simulink model "speed_control_for_IM"  (R2021a)
settings: Solver=VariableStepAuto  StartTime=0.0  StopTime=inf  MaxStep=1e-3  RelTol=1e-3
libraries: spsIGBTDiodeLib x6, spsAsynchronousMachineSIUnitsLib x1, pid_lib x1, spsDCVoltageSourceLib x1, simulink x1, spspowerguiLib x1
settings Model: Creator=AHMED  LastModifiedBy=AHMED

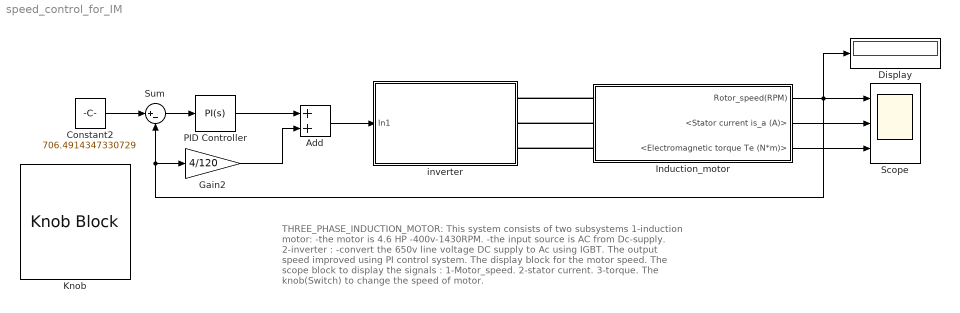
== system speed_control_for_IM ==
  note: THREE_PHASE_INDUCTION_MOTOR:
      |
      | This system consists of two subsystems
      | 1-induction motor:
      | -the motor is 4.6 HP -400v-1430RPM.
      | -the input source is AC from Dc-supply.
      | 2-inverter :
      | -convert the 650v line voltage DC supply to Ac using IGBT.
      |
      | The output speed improved using PI control system.
      | The display block for the motor speed.
      | The scope block to display the signals :
      | 1-Motor_speed.
      | 2-stator current.
      | 3-torque.
      | The knob(Switch) to change the speed of motor.
  Add : Sum
  Constant2 : Constant  Value=706.4914347330729
  Display : Display
  Gain2 : Gain  Gain=4/120
  Induction_motor : Subsystem
  Knob : KnobBlock  ScaleMax=1400
  PID Controller : pid_lib/PID Controller  Controller=PI  Form=Parallel  TimeDomain=Continuous-time  UseExternalTs=off  SampleTime=-1  IntegratorMethod=Forward Euler  FilterMethod=Forward Euler  ControllerParametersSource=internal  P=1.5  I=0.001  D=0  UseFilter=on  N=100  TunerSelectOption=Transfer Function Based (PID Tuner App)  InitialConditionSource=internal  InitialConditionForIntegrator=0  InitialConditionForFilter=0  DifferentiatorICPrevScaledInput=0  ExternalReset=none  TrackingMode=off  Kt=1  LimitOutput=on  SatLimitsSource=internal  UpperSaturationLimit=50  LowerSaturationLimit=-50  LinearizeAsGain=on  AntiWindupMode=clamping  Kb=1  POutMin=[]  POutMax=[]  IOutMin=[]  IOutMax=[]  DOutMin=[]  DOutMax=[]  NOutMin=[]  NOutMax=[]  SumOutMin=[]  SumOutMax=[]  SaturationOutMin=[]  SaturationOutMax=[]  PParamMin=[]  PParamMax=[]  IParamMin=[]  IParamMax=[]  DParamMin=[]  DParamMax=[]  NParamMin=[]  NParamMax=[]  KbParamMin=[]  KbParamMax=[]  KtParamMin=[]  KtParamMax=[]  KbOutMin=[]  KbOutMax=[]  KtOutMin=[]  KtOutMax=[]  IntegratorOutMin=[]  IntegratorOutMax=[]  FilterOutMin=[]  FilterOutMax=[]  SumI1OutMin=[]  SumI1OutMax=[]  SumI2OutMin=[]  SumI2OutMax=[]  SumI3OutMin=[]  SumI3OutMax=[]  SumI4OutMin=[]  SumI4OutMax=[]  SumDOutMin=[]  SumDOutMax=[]  DifferentiatorOutMin=[]  DifferentiatorOutMax=[]  FilterDiffOutCoefMin=[]  FilterDiffOutCoefMax=[]  ReciprocalOutMin=[]  ReciprocalOutMax=[]  SumDenOutMin=[]  SumDenOutMax=[]  SumNumOutMin=[]  SumNumOutMax=[]  DivideOutMin=[]  DivideOutMax=[]  UdiffTsProdOutMin=[]  UdiffTsProdOutMax=[]  NTsProdOutMin=[]  NTsProdOutMax=[]  UintegralTsProdOutMin=[]  UintegralTsProdOutMax=[]  UngainTsProdOutMin=[]  UngainTsProdOutMax=[]  IntegratorContinuousStateAttributes=''  IntegratorStateMustResolveToSignalObject=off  IntegratorRTWStateStorageClass=Auto  FilterContinuousStateAttributes=''  FilterStateMustResolveToSignalObject=off  FilterRTWStateStorageClass=Auto  ParallelPVariant=InternalParameters  IdealPVariant=Disabled  IVariant=InternalParameters  DVariant=Disabled  IntegratorVariant=Continuous  SatVariant=Enabled  AWVariant=ContClampingParallel  PCopyVariant=Disabled  TRVariant=Disabled  FdbkBlocksVariant=Forward  IdealPFdbkVariant=Disabled  SatFdbkVariant=Disabled  DerivativeFilterVariant=Disabled  NVariant=Disabled  NCopyVariant=Disabled_SignalSpec  FilterICVariant=Disabled  IntegratorICVariant=InternalICs  ExternalResetVariant=Disabled  TRSumVariant=Passthrough  SumFdbkVariant=Disabled  SumVariant=Sum_PI  TsampFilterVariant=InternalTs  TsampNgainVariant=Passthrough  TsampIntegralVariant=Passthrough  ExternalSaturationOutDataTypeStr=Inherit: Same as second input
  Scope : Scope  NumInputPorts=3
  Sum : Sum  Inputs=|+-
  inverter : Subsystem
  wires:
  Sum/1 -> PID Controller/1
  Constant2/1 -> Sum/1
  PID Controller/1 -> Add/1
  Gain2/1 -> Add/2
  Induction_motor/1(Rotor_speed(RPM)) -> Gain2/1, Sum/2, Scope/1, Display/1
  Induction_motor/2(<Stator current is_a (A)>) -> Scope/2
  Induction_motor/3(<Electromagnetic torque Te (N*m)>) -> Scope/3
  Add/1 -> inverter/1(In1)
  connections:
  Induction_motor/LConn1 -- inverter/RConn1
  Induction_motor/LConn2 -- inverter/RConn2
  Induction_motor/LConn3 -- inverter/RConn3

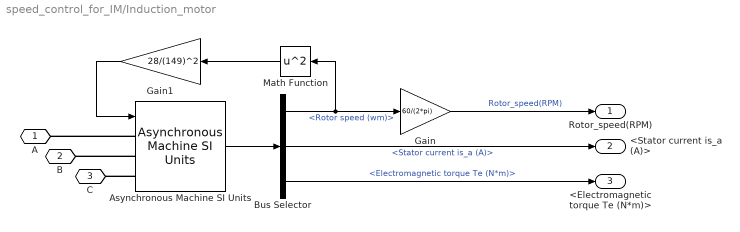
== system speed_control_for_IM/Induction_motor ==
  Asynchronous Machine SI Units : spsAsynchronousMachineSIUnitsLib/Asynchronous Machine SI Units  RotorType=Squirrel-cage  PresetModel="15:  5.4 HP (4KW)   400 V  50Hz 1430 RPM"  MechanicalLoad=Torque Tm  ShowDetailedParameters=on  ReferenceFrame=Rotor  Units=SI  MeasurementBus=off  NominalParameters=[4000 400 50]  VoltageRatio=1  Stator=[1.405 0.005839]  Rotor=[1.395 0.005839]  Cage1=[0.4155 0.002066]  Cage2=[0.4168 0.0003495]  Lm=0.1722  Mechanical=[0.0131 0.002985 2]  PolePairs=2  InitialConditions=[1 0 0 0 0 0 0 0]  SimulateSaturation=off  Saturation=[14.03593122, 27.81365428, 53.79336849, 72.68890987, 97.98006896, 148.6815601, 215.7428561, 302.9841135, 428.7778367 ; 230, 322, 414, 460, 506, 552, 598, 644, 690]  LoadFlowParameters=1492000  TsPowergui=0  TsBlock=-1  IterativeModel=Trapezoidal non iterative  IterativeDiscreteModel=Trapezoidal non iterative  Pmec=1.492e+006
  Bus Selector : BusSelector  OutputSignals=Mechanical.Rotor speed (wm),Stator measurements.Stator current is_a (A),Mechanical.Electromagnetic torque Te (N*m)
  Gain : Gain  Gain=60/(2*pi)
  Gain1 : Gain  Gain=28/(149)^2
  Math Function : Math  Operator=square  SaturateOnIntegerOverflow=on
  A : PMIOPort  Side=Left
  B : PMIOPort  Port=2  Side=Left
  C : PMIOPort  Port=3  Side=Left
  Rotor_speed(RPM) : Outport
  <Stator current is_a (A)> : Outport  Port=2
  <Electromagnetic torque Te (N*m)> : Outport  Port=3
  wires:
  Gain/1 -> Rotor_speed(RPM)/1  "Rotor_speed(RPM)"
  Bus Selector/1 -> Math Function/1, Gain/1  "<Rotor speed (wm)>"
  Bus Selector/3 -> <Electromagnetic torque Te (N*m)>/1  "<Electromagnetic torque Te (N*m)>"
  Bus Selector/2 -> <Stator current is_a (A)>/1  "<Stator current is_a (A)>"
  Asynchronous Machine SI Units/1 -> Bus Selector/1
  Gain1/1 -> Asynchronous Machine SI Units/1
  Math Function/1 -> Gain1/1
  connections:
  Asynchronous Machine SI Units/LConn1 -- A/RConn1
  Asynchronous Machine SI Units/LConn2 -- B/RConn1
  Asynchronous Machine SI Units/LConn3 -- C/RConn1

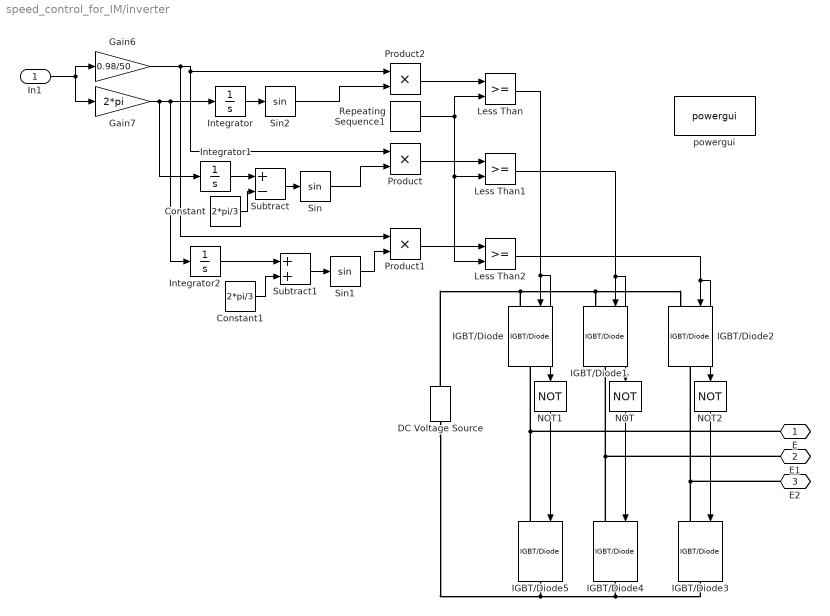
== system speed_control_for_IM/inverter ==
  In1 : Inport
  Constant : Constant  Value=2*pi/3
  Constant1 : Constant  Value=2*pi/3
  DC Voltage Source : spsDCVoltageSourceLib/DC Voltage Source  Amplitude=650  Measurements=None
  Gain6 : Gain  Gain=0.98/50
  Gain7 : Gain  Gain=2*pi
  IGBT/Diode{,1..5} (6 alike) : spsIGBTDiodeLib/IGBT//Diode  Ron=1e-3  Rs=1e5  Cs=inf  Measurements=off
  Integrator : Integrator
  Integrator1 : Integrator
  Integrator2 : Integrator
  Less Than : RelationalOperator  OutDataTypeStr=boolean  RndMeth=Simplest
  Less Than1 : RelationalOperator  OutDataTypeStr=boolean  RndMeth=Simplest
  Less Than2 : RelationalOperator  OutDataTypeStr=boolean  RndMeth=Simplest
  NOT : Logic  Operator=NOT  AllPortsSameDT=off  OutDataTypeStr=boolean
  NOT1 : Logic  Operator=NOT  AllPortsSameDT=off  OutDataTypeStr=boolean
  NOT2 : Logic  Operator=NOT  AllPortsSameDT=off  OutDataTypeStr=boolean
  Product : Product
  Product1 : Product
  Product2 : Product
  Repeating Sequence1 : simulink/Sources/Repeating Sequence  rep_seq_t=[0 (1/5000)/4 (1/5000)/2 (3/5000)/4 1/5000]  rep_seq_y=[0 1 0 -1 0]
  Sin : Trigonometry
  Sin1 : Trigonometry
  Sin2 : Trigonometry
  Subtract : Sum  Inputs=+-
  Subtract1 : Sum
  powergui : spspowerguiLib/powergui  Priority=1  SimulationMode=Discrete  SampleTime=1e-6  frequency=60  Iterations=50  frequencyindice=50  Pbase=100e6  ErrMax=1e-4  UnitsV=kV  UnitsW=MW  buscounter=0  FunctionMessages=off  echomessages=off  EnableUseOfTLC=off  CurrentSourceSwitches=off  DisableSnubberDevices=off  DisableRonSwitches=off  DisableVfSwitches=off  DisplayEquations=off  AutomaticDiscreteSolvers=off  SolverType=Tustin/Backward Euler (TBE)  Interpol=off  ExternalGateDelay=off  methode=off  Ts=100  x0status=blocks  SPID=on  SwTol=0  HookPort=off  NonlinearTolerance=1e-4  nMaxIteration=100  ContinueOnMaxIteration=off  RestoreLinks=warning  ResistiveCurrentMeasurement=off  Frange=[0:2:500]  Ylog=off  Xlog=on  ShowGrid=off  save=off  variable=ZData  structure=0  ZoomFFT=off  StartTime=0.0  cycles=1  DisplayStyle=1  fundamental=60  FreqAxis=off  MaxFrequency=1000  frequencyindicesteady=1  RmsSteady=1  display=off
  E : PMIOPort  Side=Right
  E1 : PMIOPort  Port=2  Side=Right
  E2 : PMIOPort  Port=3  Side=Right
  wires:
  NOT/1 -> IGBT/Diode4/1
  Subtract1/1 -> Sin1/1
  In1/1 -> Gain6/1, Gain7/1
  NOT1/1 -> IGBT/Diode5/1
  Integrator2/1 -> Subtract1/1
  Less Than1/1 -> NOT/1, IGBT/Diode1/1
  Gain6/1 -> Product1/1, Product/1, Product2/1
  NOT2/1 -> IGBT/Diode3/1
  Less Than/1 -> NOT1/1, IGBT/Diode/1
  Subtract/1 -> Sin/1
  Sin/1 -> Product/2
  Less Than2/1 -> NOT2/1, IGBT/Diode2/1
  Integrator1/1 -> Subtract/1
  Integrator/1 -> Sin2/1
  Constant1/1 -> Subtract1/2
  Repeating Sequence1/1 -> Less Than1/2, Less Than2/2, Less Than/2
  Product1/1 -> Less Than2/1
  Product2/1 -> Less Than/1
  Gain7/1 -> Integrator1/1, Integrator2/1, Integrator/1
  Product/1 -> Less Than1/1
  Sin2/1 -> Product2/2
  Sin1/1 -> Product1/2
  Constant/1 -> Subtract/2
  connections:
  IGBT/Diode5/RConn1 -- DC Voltage Source/LConn1 -- IGBT/Diode3/RConn1 -- IGBT/Diode4/RConn1
  IGBT/Diode/LConn1 -- DC Voltage Source/RConn1 -- IGBT/Diode2/LConn1 -- IGBT/Diode1/LConn1
  IGBT/Diode4/LConn1 -- IGBT/Diode1/RConn1 -- E1/RConn1
  IGBT/Diode5/LConn1 -- IGBT/Diode/RConn1 -- E/RConn1
  IGBT/Diode3/LConn1 -- IGBT/Diode2/RConn1 -- E2/RConn1
